simulink model "QUESTION1C"  (R2021b)
settings: Solver=VariableStepAuto  StartTime=0.0  StopTime=10.0  RelTol=1e-3
settings Model: Creator=Progg  LastModifiedBy=Progg

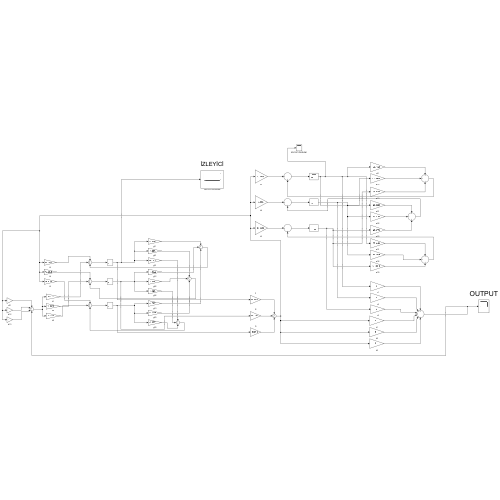
[thumbnail: Simulink's stored preview of the top-level diagram]
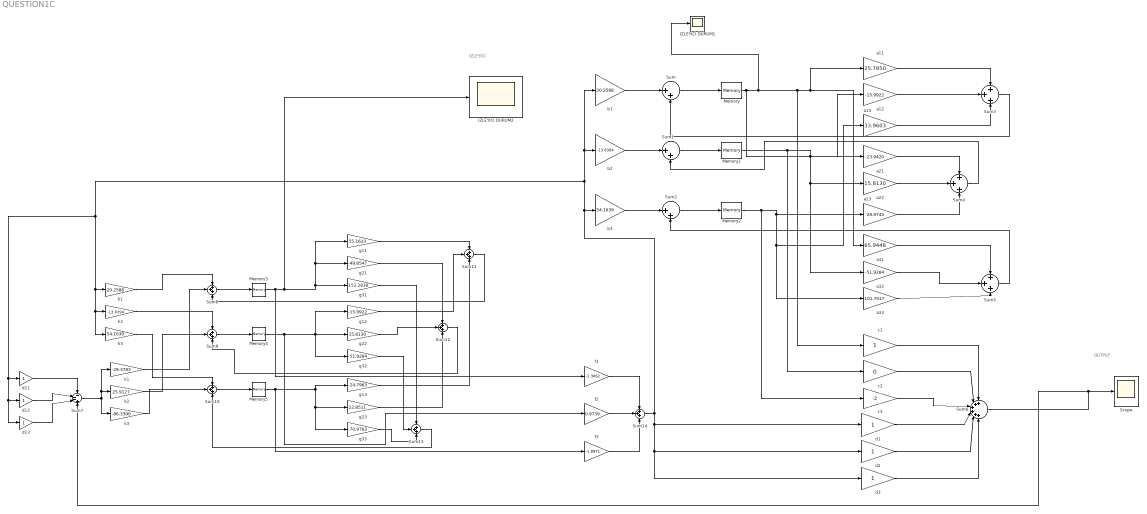
== system QUESTION1C ==
  note: OUTPUT
  note: İZLEYİCİ
  IZLEYICI DURUM1 : Scope
  IZLEYICI DURUM2 : Scope
  Memory{,1..5} (6 alike) : Memory  InitialCondition=5
  Scope : Scope
  Sum : Sum  Inputs=|++
  Sum1 : Sum  Inputs=|++
  Sum{3..5,8..14} (10 alike) : Sum  Inputs=+++
  Sum2 : Sum  Inputs=|++
  Sum6 : Sum  Inputs=++++++
  Sum7 : Sum  Inputs=---+
  a11 : Gain  Gain=25.7850
  a12 : Gain  Gain=-15.9922
  a13 : Gain  Gain=33.9603
  a21 : Gain  Gain=-23.9420
  a22 : Gain  Gain=15.8130
  a23 : Gain  Gain=-28.9743
  a31 : Gain  Gain=65.9448
  a32 : Gain  Gain=-51.9284
  a33 : Gain  Gain=101.7017
  b1 : Gain  Gain=20.2588
  b2 : Gain  Gain=-13.6394
  b3 : Gain  Gain=54.1639
  c1 : Gain
  c2 : Gain  Gain=0
  c3 : Gain  Gain=-2
  d{1..3,11..13} (6 alike) : Gain
  f1 : Gain  Gain=-1.3062
  f2 : Gain  Gain=0.9739
  f3 : Gain  Gain=-1.8971
  g11 : Gain  Gain=55.1633
  g12 : Gain  Gain=-15.9922
  g13 : Gain  Gain=-24.7963
  g21 : Gain  Gain=-49.8547
  g22 : Gain  Gain=15.8130
  g23 : Gain  Gain=22.8511
  g31 : Gain  Gain=152.2838
  g32 : Gain  Gain=-51.9284
  g33 : Gain  Gain=-70.9763
  h1 : Gain  Gain=20.2588
  h2 : Gain  Gain=-13.6394
  h3 : Gain  Gain=54.1639
  k1 : Gain  Gain=-29.3783
  k2 : Gain  Gain=25.9127
  k3 : Gain  Gain=-86.3390
  wires:
  d11/1 -> Sum7/1
  d12/1 -> Sum7/2
  d13/1 -> Sum7/3
  Sum7/1 -> k2/1, k1/1, k3/1
  h1/1 -> Sum8/1
  k1/1 -> Sum8/2
  h2/1 -> Sum9/1
  k2/1 -> Sum9/2
  h3/1 -> Sum10/1
  k3/1 -> Sum10/2
  Sum8/1 -> Memory3/1
  Sum9/1 -> Memory4/1
  Sum10/1 -> Memory5/1
  Memory3/1 -> f1/1, IZLEYICI DURUM2/1, g21/1, g11/1, g31/1
  Memory4/1 -> f2/1, g12/1, g32/1, g22/1
  Memory5/1 -> f3/1, g13/1, g33/1, g23/1
  d2/1 -> Sum6/5
  d1/1 -> Sum6/4
  c2/1 -> Sum6/2
  b2/1 -> Sum1/1
  d3/1 -> Sum6/6
  c1/1 -> Sum6/1
  Sum3/1 -> Sum/2
  Sum1/1 -> Memory1/1
  Sum4/1 -> Sum1/2
  a21/1 -> Sum4/1
  Sum5/1 -> Sum2/2
  a13/1 -> Sum3/3
  a31/1 -> Sum5/1
  b1/1 -> Sum/1
  a12/1 -> Sum3/2
  a11/1 -> Sum3/1
  Sum6/1 -> Sum7/4, Scope/1
  a32/1 -> Sum5/2
  a33/1 -> Sum5/3
  a23/1 -> Sum4/3
  b3/1 -> Sum2/1
  Memory2/1 -> c3/1, a33/1, a13/1, a23/1
  Memory1/1 -> c2/1, a32/1, a22/1, a12/1
  a22/1 -> Sum4/2
  Sum/1 -> Memory/1
  Memory/1 -> a21/1, IZLEYICI DURUM1/1, c1/1, a11/1, a31/1
  Sum2/1 -> Memory2/1
  c3/1 -> Sum6/3
  g11/1 -> Sum11/1
  g12/1 -> Sum11/2
  g13/1 -> Sum11/3
  Sum11/1 -> Sum8/3
  g21/1 -> Sum12/1
  g22/1 -> Sum12/2
  g23/1 -> Sum12/3
  Sum12/1 -> Sum9/3
  g33/1 -> Sum13/3
  g32/1 -> Sum13/2
  g31/1 -> Sum13/1
  Sum13/1 -> Sum10/3
  f2/1 -> Sum14/2
  f1/1 -> Sum14/1
  f3/1 -> Sum14/3
  Sum14/1 -> d3/1, d2/1, d1/1, d13/1, d12/1, d11/1, h3/1, h2/1, h1/1, b1/1, b2/1, b3/1
